simulink model "model1"  (R2024a)
settings: Solver=VariableStepAuto  StartTime=0.0  StopTime=10  RelTol=1e-8
values from neighbouring files (symbols this model uses):
  a0 = 57.41    [script1.m]    (also in script11.m; script12.m = 361; sctipt13.m = 49.81)
  a1 = 5.8    [script1.m]    (also in script11.m; script12.m = 0; sctipt13.m = -1.8)
  dy0 = 0    [script1.m]    (also in script11.m; script12.m; sctipt13.m)
  y0 = y0_values(i)    [script1.m]    (also in script11.m; script12.m; sctipt13.m)
settings Model: Creator=eva  LastModifiedBy=eva

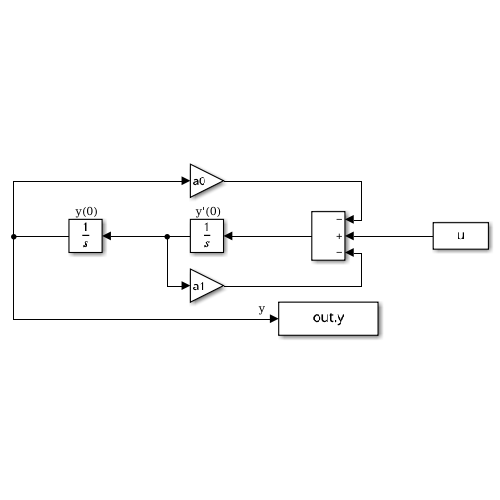
[thumbnail: Simulink's stored preview of the top-level diagram]
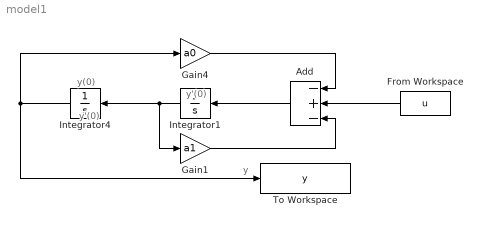
== system model1 ==
  note: y
  note: y'(0)
  note: y'(0)
  note: y(0)
  Add : Sum  Inputs=-+-
  From Workspace : FromWorkspace  VariableName=u
  Gain1 : Gain  Gain=a1
  Gain4 : Gain  Gain=a0
  Integrator1 : Integrator  InitialCondition=dy0
  Integrator4 : Integrator  InitialCondition=y0
  To Workspace : ToWorkspace  VariableName=y  SaveFormat=Structure With Time  SampleTime=-1
  wires:
  Integrator1/1 -> Gain1/1, Integrator4/1
  Integrator4/1 -> To Workspace/1, Gain4/1
  Add/1 -> Integrator1/1
  Gain4/1 -> Add/1
  Gain1/1 -> Add/3
  From Workspace/1 -> Add/2
